simulink model "main"  (R2020a)
settings: Solver=VariableStepAuto  StartTime=0.0  StopTime=2  RelTol=1e-3
Description:
  | 基于动力学模型补偿的机械手PD控制方法
settings Model: Creator=yuan_  LastModifiedBy=yuan_

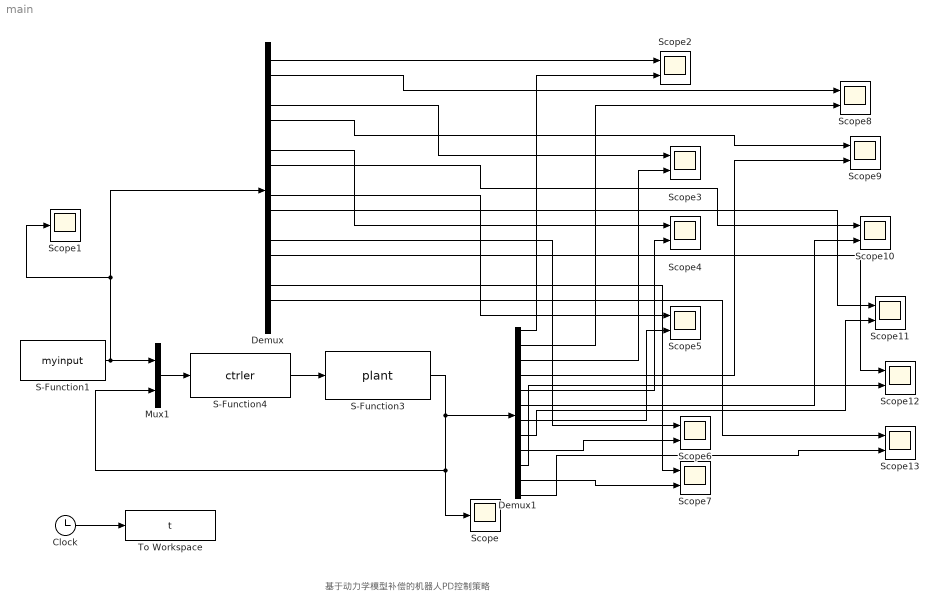
== system main ==
  note: 基于动力学模型补偿的机器人PD控制策略
  Clock : Clock
  Demux : Demux  Outputs=18
  Demux1 : Demux  Outputs=12
  Mux1 : Mux  Inputs=2
  S-Function1 : S-Function  FunctionName=myinput  SFunctionDeploymentMode=off  EnableBusSupport=off
  S-Function3 : S-Function  FunctionName=plant  SFunctionDeploymentMode=off  EnableBusSupport=off
  S-Function4 : S-Function  FunctionName=ctrler  SFunctionDeploymentMode=off  EnableBusSupport=off
  Scope : Scope
  Scope1 : Scope
  Scope{2..13} (12 alike) : Scope  NumInputPorts=2
  To Workspace : ToWorkspace  VariableName=t  SaveFormat=Timeseries  SampleTime=-1
  wires:
  S-Function1/1 -> Demux/1, Scope1/1, Mux1/1
  S-Function4/1 -> S-Function3/1
  Mux1/1 -> S-Function4/1
  S-Function3/1 -> Scope/1, Mux1/2, Demux1/1
  Clock/1 -> To Workspace/1
  Demux/1 -> Scope2/1
  Demux1/1 -> Scope2/2
  Demux/4 -> Scope3/1
  Demux1/3 -> Scope3/2
  Demux1/5 -> Scope4/2
  Demux1/7 -> Scope5/2
  Demux1/9 -> Scope6/2
  Demux1/11 -> Scope7/2
  Demux/7 -> Scope4/1
  Demux/10 -> Scope5/1
  Demux/13 -> Scope6/1
  Demux/16 -> Scope7/1
  Demux/2 -> Scope8/1
  Demux1/2 -> Scope8/2
  Demux/5 -> Scope9/1
  Demux1/4 -> Scope9/2
  Demux/8 -> Scope10/1
  Demux1/6 -> Scope10/2
  Demux/11 -> Scope11/1
  Demux1/8 -> Scope11/2
  Demux/14 -> Scope12/1
  Demux1/10 -> Scope12/2
  Demux/17 -> Scope13/1
  Demux1/12 -> Scope13/2
